simulink model "HeartModel"  (R2014a)
settings: Solver=FixedStepDiscrete  StartTime=0.0  StopTime=100  FixedStep=0.01  RelTol=1e-3
settings Model: Creator=alexandru  LastModifiedBy=barbot
settings DataIOCC: LimitDataPoints=off  SaveOutput=off  SignalLogging=off  DSMLogging=off  SaveTime=off
settings HardwareCC: TargetBitPerLong=64  TargetBitPerPointer=64  TargetLongLongMode=on  TargetIntDivRoundTo=Zero  TargetEndianess=LittleEndian  TargetWordSize=64  TargetHWDeviceType=MATLAB Host  ProdEqTarget=off
settings RTWCC: SystemTargetFile=rsim.tlc  GenCodeOnly=on  PackageGeneratedCodeAndArtifacts=on  PackageName=idhp_model_heart_realtime  TemplateMakefile=rsim_default_tmf  Description=Rapid Simulation Target  ProcessScript=rsim_make_rtw_hook
settings RSimTargetCC: ERTMultiwordTypeDef=System defined  ERTMultiwordLength=256  EnableShiftOperators=on

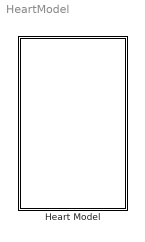
== system HeartModel ==
  Heart Model : Stateflow chart  Priority=1  TreatAsAtomicUnit=on

== stateflow chart HeartModel/Heart Model ==
  state Heart
    state A_dV [parallel]
      settings: executionOrder=13
      state a_dVLow
      state a_dvHigh
      (default) -> a_dVLow
      a_dVLow -> a_dvHigh [order 1] : a_dVSetHigh
      a_dVLow -> a_dVLow [order 2] : tr_AVJ
          | {send(AVJAnteReached,AVJ);}
      a_dvHigh -> a_dvHigh [order 2] : tr_AVJ
          | {send(AVJAnteReachedHigh,AVJ);}
      a_dvHigh -> a_dVLow [order 1] : a_dVSetLow
    state AVJOut [parallel]
      settings: executionOrder=4
      state Empty
      state Ante
      state Retro
      (default) -> Heart.AVJOut.Empty : {AV_alpha = 150;
          | AV_anteDMin = 50;
          | AV_retroDMin = 100;
          | AV_tauC = 100;
          | }
      Heart.AVJOut.Ante -> Heart.AVJOut.Empty : after(AVJDelay(avj_tRec,...
          | AV_anteDMin),msec)
          | {send(anteAVJ,RVConductor);}
      Heart.AVJOut.Empty -> Heart.AVJOut.Ante [order 1] : AVJAnteExit
      Heart.AVJOut.Retro -> Heart.AVJOut.Empty : after(AVJDelay(avj_tRec,...
          | AV_retroDMin),msec)
          | {send(retroAVJ,...
          | RAConductor);}
      Heart.AVJOut.Empty -> Heart.AVJOut.Retro [order 2] : AVJRetroExit
    state VRGEctopic [parallel]
      settings: executionOrder=10
      state q0
      (default) -> Heart.VRGEctopic.q0 : {VRG_ectopD = 30450;}
      Heart.VRGEctopic.q0 -> Heart.VRGEctopic.q0 : after(VRG_ectopD, msec)
          | {send(Vbeat,Ventricle);}
    state VtrNoiseGenerator [parallel]
      settings: executionOrder=3
      state q0
      (default) -> Heart.VtrNoiseGenerator.q0 : {VRG_noiseD = 1000000;}
      Heart.VtrNoiseGenerator.q0 -> Heart.VtrNoiseGenerator.q0 : after(VRG_noiseD, msec)
    state RVConductor [parallel]
      settings: executionOrder=5
      state Empty
      state Ante
      state Retro
      (default) -> Heart.RVConductor.Empty : {RV_anteD = 50;
          | RV_retroD = 50;}
      Heart.RVConductor.Empty -> Heart.RVConductor.Ante [order 1] : anteAVJ
      Heart.RVConductor.Empty -> Heart.RVConductor.Retro [order 2] : vrg
      Heart.RVConductor.Ante -> Heart.RVConductor.Empty [order 1] : vrg
      Heart.RVConductor.Ante -> Heart.RVConductor.Empty [order 2] : after(RV_anteD,msec)
          | {send(VtrAnteReached,...
          | Ventricle);}
      Heart.RVConductor.Retro -> Heart.RVConductor.Empty [order 1] : anteAVJ
      Heart.RVConductor.Retro -> Heart.RVConductor.Empty [order 2] : after(RV_retroD,msec)
          | {send(AVJRetroReached,...
          | AVJ);}
    state RAConductor [parallel]
      settings: executionOrder=6
      state Empty
      state Ante
      state Retro
      (default) -> Heart.RAConductor.Empty : {RA_anteD = 30;
          | RA_retroD = 30;}
      Heart.RAConductor.Empty -> Heart.RAConductor.Ante [order 1] : arg
      Heart.RAConductor.Ante -> Heart.RAConductor.Empty [order 1] : retroAVJ
      Heart.RAConductor.Empty -> Heart.RAConductor.Retro [order 2] : retroAVJ
      Heart.RAConductor.Retro -> Heart.RAConductor.Empty [order 1] : arg
      Heart.RAConductor.Retro -> Heart.RAConductor.Empty [order 2] : after(RA_retroD,msec)
          | {send(AtrRetroReached,...
          | Atrium);}
      Heart.RAConductor.Ante -> Heart.RAConductor.Empty [order 2] : after(RA_anteD,msec)
          | {send(tr_AVJ,A_dV);}
    state SANodeEctopic [parallel]
      settings: executionOrder=2
      state q0
      (default) -> Heart.SANodeEctopic.q0 : {SA_ectopD = 10400;}
      Heart.SANodeEctopic.q0 -> Heart.SANodeEctopic.q0 : after(SA_ectopD, msec)
          | {send(Abeat,Atrium);
          | send(a_dVSetHigh,A_dV);}
    state AtrNoiseGenerator [parallel]
      settings: executionOrder=1
      state q0
      Heart.AtrNoiseGenerator.q0 -> Heart.AtrNoiseGenerator.q0 : after(SA_noiseD, msec)
      (default) -> Heart.AtrNoiseGenerator.q0 : {SA_noiseD = 1000000;}
    state VRG [parallel]
      settings: executionOrder=11
      state Wait4VBeat
      state Wait4VSynch
      (default) -> Wait4VBeat : {VRG_d = 3000;}
      Wait4VBeat -> Wait4VSynch [order 2] : after(VRG_d, msec)
          | {send(Vbeat,Ventricle);}
      Wait4VSynch -> Wait4VBeat : NextVtrBeat
      Wait4VBeat -> Wait4VBeat [order 1] : NextVtrBeat
    state SANode [parallel]
      settings: executionOrder=7
      state Wait4ABeat
      state Wait4ASynch
      (default) -> Wait4ABeat : {SA_d = 850;}
      Wait4ABeat -> Wait4ASynch [order 2] : after(SA_d, msec)
          | {send(Abeat,Atrium);
          | send(a_dVSetLow,A_dV);
          | }
      Wait4ABeat -> Wait4ABeat [order 1] : NextAtrBeat
      Wait4ASynch -> Wait4ABeat : NextAtrBeat
    state AVJ [parallel]
      settings: executionOrder=12
      state Recovery
      state Ante
      state Refractory
      state Retro
      Heart.AVJ.Ante -> Heart.AVJ.Refractory : after(avj_t4,msec)
          | {ctime=ctime+temporalCount(msec);
          | avj_tRec=(ctime-recoverylast);
          | send(AVJAnteExit,AVJOut);
          | avj_refr_0=initRefrPeriod(avj_tRec);
          | avj_refr=avj_refr_0;
          | refractorylast=ctime;}
      Recovery -> Heart.AVJ.Ante [order 1] : AVJAnteReached{
          | ctime=ctime+temporalCount(msec);
          | avj_t4 = timeToDep(AV_Vr+ ...
          | (ctime-recoverylast)*AV_k4 + SA_dV);
          | }
      Recovery -> Heart.AVJ.Ante [order 3] : AVJAnteReachedHigh{
          | ctime=ctime+temporalCount(msec);
          | avj_t4 = timeToDep(AV_Vr+...
          | (ctime-recoverylast)*AV_k4 + SA_ectopdV);
          | }
      Heart.AVJ.Refractory -> Recovery [order 4] : after(avj_refr,msec){
          | ctime=ctime+temporalCount(msec);
          | avj_t4=timeToDep(AV_Vr);
          | recoverylast=ctime;
          | }
      (default) -> Recovery : {AV_Vr = -90;
          | AV_Vt = -40;
          | AV_beta = 250;
          | AV_delta = 10;
          | AV_k4 = 0.03;
          | AV_refrDMin = 50;
          | AV_theta = 10;
          | AV_tr = 500;
          | SA_dV = 50;
          | SA_ectopdV = 50;
          | avj_t4=timeToDep(AV_Vr);
          | ctime=0;
          | recoverylast=0;
          | refractorylast=0;
          | }
      Recovery -> Heart.AVJ.Retro [order 4] : AVJRetroReached{
          | ctime=ctime+temporalCount(msec);}
      Recovery -> Heart.AVJ.Refractory [order 2] : after(avj_t4,msec){
          | ctime=ctime+temporalCount(msec);
          | avj_tRec=avj_t4;
          | avj_refr_0=initRefrPeriod(avj_tRec);
          | avj_refr=avj_refr_0;
          | refractorylast=ctime;}
      Heart.AVJ.Refractory -> Heart.AVJ.Refractory [order 3] : AVJAnteReachedHigh
          | {ctime=ctime+temporalCount(msec);
          | avj_refr=avj_refr-(ctime - refractorylast)+...
          | modulateRefrAnte((ctime - refractorylast),...
          | avj_refr_0,SA_ectopdV);
          | refractorylast=ctime;
          | }
      Heart.AVJ.Refractory -> Heart.AVJ.Refractory [order 1] : AVJAnteReached
          | {ctime=ctime+temporalCount(msec);
          | avj_refr=avj_refr-(ctime - refractorylast)+...
          | modulateRefrAnte((ctime - refractorylast),...
          | avj_refr_0,SA_dV);
          | refractorylast=ctime;}
      Heart.AVJ.Refractory -> Heart.AVJ.Refractory [order 2] : AVJRetroReached
          | {ctime=ctime+temporalCount(msec);
          | avj_refr=avj_refr-(ctime - refractorylast)+...
          | modulateRefrRetro((ctime - refractorylast),...
          | avj_refr_0);
          | refractorylast=ctime;}
      Heart.AVJ.Retro -> Heart.AVJ.Refractory : {send(AVJRetroExit,AVJOut);
          | ctime=ctime+temporalCount(msec);
          | avj_tRec=ctime-recoverylast;
          | avj_refr_0=initRefrPeriod(avj_tRec);
          | avj_refr=avj_refr_0;
          | refractorylast=ctime;
          | }
    state Ventricle [parallel]
      settings: executionOrder=8
      state Excitable
      state Refractory
      state VsenseAnte
      state VSynch
      state Vsense
      state GenerateRetroWave
      (default) -> Heart.Ventricle.Refractory : {Vtr_refrD = 200;}
      Heart.Ventricle.Refractory -> Heart.Ventricle.Excitable : after(Vtr_refrD,msec)
      Heart.Ventricle.Excitable -> GenerateRetroWave [order 2] : VP
      Heart.Ventricle.Excitable -> Vsense [order 3] : Vbeat
      Heart.Ventricle.Excitable -> VsenseAnte [order 1] : VtrAnteReached
      VSynch -> Heart.Ventricle.Refractory : {send(NextVtrBeat,...
          | VRG);}
      VsenseAnte -> VSynch : {SWrite(0xAB, 0x32, 0x55);}
      GenerateRetroWave -> VSynch : {send(vrg,RVConductor);}
      Vsense -> GenerateRetroWave : {SWrite(0xAB, 0x32, 0x55);}
    state Atrium [parallel]
      settings: executionOrder=9
      state Excitable
      state Refractory
      state AsenseRetro
      state ASynch
      state Asense
      state GenerateAnteWave
      (default) -> Heart.Atrium.Refractory : {Atr_refrD = 50;}
      Heart.Atrium.Excitable -> Asense [order 1] : Abeat
      Heart.Atrium.Refractory -> Heart.Atrium.Excitable : after(Atr_refrD,msec)
      Heart.Atrium.Excitable -> AsenseRetro [order 3] : AtrRetroReached
      ASynch -> Heart.Atrium.Refractory : {send(NextAtrBeat,...
          | SANode);}
      Heart.Atrium.Excitable -> GenerateAnteWave [order 2] : AP
      AsenseRetro -> ASynch : {SWrite(0xAB, 0x31, 0x55);}
      GenerateAnteWave -> ASynch : {send(arg,RAConductor);}
      Asense -> GenerateAnteWave : {SWrite(0xAB, 0x31, 0x55);}
    state Parameter_Serial [parallel]
      settings: executionOrder=15
      state Init
      state DataReceived
      state Data
      state EndHeader
      state CHeader
      state DataParId1
      state DataParId2
      state DataParValue1
      state DataParValue2
      state DataParValue3
      state DataParValue4
      state HeaderPar
      state CHeaderPar
      CHeader -> Init [order 3] : [bufs1==0x04 && bufs2==0x55]
          | {send(VP, Ventricle);}
      DataReceived -> Init [order 2] : [bufs1!=0xAB || bufs1!=0xAA]
      Init -> DataReceived : SREC
          | {bufs1 = SReceive();}
      EndHeader -> CHeader : SREC
          | {bufs2 = SReceive();}
      Data -> EndHeader : SREC
          | {bufs1 = SReceive();}
      DataReceived -> Data [order 1] : [bufs1==0xAB]
      (default) -> Init : {BAUDRATE = 115200;}
      CHeaderPar -> Init [order 2] : [bufs5==0x55]
          | {SetParameter(parid, parval);}
      CHeaderPar -> Init [order 1] : [bufs5!=0x55]
      CHeader -> Init [order 2] : [bufs1==0x03 && bufs2==0x55]
          | {send(AP, Atrium);}
      CHeader -> Init [order 1] : [bufs2!=0x55 || (bufs1!=0x03 && bufs1!=0x04)]
      DataReceived -> DataParId1 [order 3] : [bufs1==0xAA]
      DataParValue2 -> DataParValue3 : SREC
          | {bufs2= SReceive();}
      DataParValue1 -> DataParValue2 : SREC
          | {bufs1 = SReceive();}
      DataParId2 -> DataParValue1 : SREC
          | {bufs2= SReceive();
          | tmp16 = bufs2;
          | parid=(tmp16<<8) | bufs1;}
      DataParValue3 -> DataParValue4 : SREC
          | {bufs3= SReceive();}
      DataParId1 -> DataParId2 : SREC
          | {bufs1= SReceive();}
      DataParValue4 -> HeaderPar : SREC
          | {bufs4 = SReceive();
          | tmp32 = bufs4;
          | value = tmp32<<24;
          | tmp32 = bufs3;
          | value = value | (tmp32<<16);
          | tmp32 = bufs2;
          | value = value | (tmp32<<8);
          | value = value | bufs1;
          | parval = ConvertIntToDouble(value);}
      HeaderPar -> CHeaderPar : SREC
          | {bufs5 = SReceive();}
    state SerialPort [parallel]
      settings: executionOrder=14
      state NoData
      state DataAvailable
      (default) -> NoData
      DataAvailable -> NoData : {send(SREC,Parameter_Serial);}
  (default) -> Heart
  data: t function_output double; tRec function_input double; minDly function_input double; t function_output double; Vm function_input double; t function_input double; t0 function_input double; dT function_output double; dV function_input double; t function_input double; dT function_output double; t0 function_input double; t function_output double; tRec function_input double; buf function_output double; stat function_output double; parid function_input double; parval function_input double; value function_input double; parval function_output double; stat function_output double; h function_input double; d function_input double; e function_input double; Atr_refrD local double; AV_alpha local double; AV_anteDMin local double; AV_beta local double; AV_delta local double; AV_k4 local double; AV_refrDMin local double; AV_retroDMin local double; AV_tauC local double; AV_theta local double; AV_tr local double; AV_Vr local double; AV_Vt local double; RA_anteD local double; RA_retroD local double; RV_anteD local double; RV_retroD local double; SA_d local double; SA_dV local double; SA_ectopD local double; SA_ectopdV local double; SA_noiseD local double; VRG_d local double; VRG_ectopD local double; VRG_noiseD local double; Vtr_refrD local double; avj_tRec local double; clk local double; recoverylast local double; avj_t4 local double; ctime local double; avj_refr local double; avj_refr_0 local double; refractorylast local double; BAUDRATE local uint32; bufs1 local uint8; bufs2 local uint8; bufs3 local uint8; bufs4 local uint8; bufs5 local uint8; parid local uint16; value local uint32; parval local double; tmp16 local uint16; tmp32 local uint32
  events: Abeat local FUNCTION_CALL_EVENT; AtrRetroReached local FUNCTION_CALL_EVENT; arg local FUNCTION_CALL_EVENT; retroAVJ local FUNCTION_CALL_EVENT; AVJAnteReached local FUNCTION_CALL_EVENT; NextAtrBeat local FUNCTION_CALL_EVENT; AVJRetroReached local FUNCTION_CALL_EVENT; anteAVJ local FUNCTION_CALL_EVENT; vrg local FUNCTION_CALL_EVENT; VtrAnteReached local FUNCTION_CALL_EVENT; AVJRetroExit local FUNCTION_CALL_EVENT; AVJAnteExit local FUNCTION_CALL_EVENT; NextVtrBeat local FUNCTION_CALL_EVENT; Vbeat local FUNCTION_CALL_EVENT; AP local EITHER_EDGE_EVENT; VP local EITHER_EDGE_EVENT; AS local RISING_EDGE_EVENT; VS local RISING_EDGE_EVENT; Aget local EITHER_EDGE_EVENT; Vget local EITHER_EDGE_EVENT; Aintrinsic local EITHER_EDGE_EVENT; Anoise local EITHER_EDGE_EVENT; Aretro local EITHER_EDGE_EVENT; Vintrinsic local EITHER_EDGE_EVENT; Vnoise local EITHER_EDGE_EVENT; APElectr local RISING_EDGE_EVENT; VPElectr local EITHER_EDGE_EVENT; IncrClk local FUNCTION_CALL_EVENT; State local FUNCTION_CALL_EVENT; Clk0 local FUNCTION_CALL_EVENT; Clk1 local FUNCTION_CALL_EVENT; a_dVSetHigh local FUNCTION_CALL_EVENT; a_dVSetLow local FUNCTION_CALL_EVENT; tr_AVJ local FUNCTION_CALL_EVENT; AVJAnteReachedHigh local FUNCTION_CALL_EVENT; RLRI local FUNCTION_CALL_EVENT; TAVI local FUNCTION_CALL_EVENT; RTAVI local FUNCTION_CALL_EVENT; RURI local FUNCTION_CALL_EVENT; SREC local FUNCTION_CALL_EVENT
  function t  = AVJDelay(tRec,minDly):
    | function t  = AVJDelay(tRec,minDly)
    |     t = minDly+AV_alpha*exp(-tRec/AV_tauC);
    | end
  function t  = timeToDep(Vm):
    | function t  = timeToDep(Vm)
    |     t = max(0,(AV_Vt-Vm)/AV_k4);
    | end
  function dT  = modulateRefrAnte(t,t0,dV):
    | function dT  = modulateRefrAnte(t,t0,dV)
    |     %val1 = t/t0;
    |     %val2 = power(t/t0,avj_theta);
    |     dT = AV_refrDMin*power(t/t0,AV_theta)*power(min(1,dV/(AV_Vt-AV_Vr)),AV_delta);
    |     %fprintf(1,'%f %f\n', val1, val2);
    | end
  function dT  = modulateRefrRetro(t,t0):
    | 
    | function dT  = modulateRefrRetro(t,t0)
    |     dT = AV_refrDMin*power(t/t0,AV_theta);
    | end
  function t  = initRefrPeriod(tRec):
    | function t  = initRefrPeriod(tRec)
    |     t = AV_refrDMin + AV_beta*(1 - exp(-tRec/AV_tr));
    | end
  function buf  = SReceive:
    | function buf  = SReceive()
    |     buf = 0;
    | end
  function stat  = SetParameter(parid, parval):
    | function stat  = SetParameter(parid, parval)
    |     stat = 0;
    |     if (parid==1) 
    |         SA_d = parval;
    |         return;
    |     end
    | 
    |     if (parid==2) 
    |         SA_noiseD = parval;
    |         return;
    |     end
    | 
    |     if (parid==3) 
    |         SA_ectopD = parval;
    |         return;
    |     end
    |     
    |     return;
    | end
  function parval  = ConvertIntToDouble(value):
    | function parval  = ConvertIntToDouble(value)
    |     parval = 0;
    | end
  function stat  = SWrite(h,d,e):
    | function stat  = SWrite(h,d,e)
    | stat = 0;
    | end
